simulink model "Servosistema_integrador_realimentacao"  (R2023b)
settings: Solver=FixedStepAuto  StartTime=0.0  StopTime=5  FixedStep=T  RelTol=1e-3
model workspace (MAT data in the model file):
  B = 0.0928995746863
  J = 0.56
  K = [0.48 -97.1871]
  Kf = 1.9158692362
  Ki = -97.6271
  Ko = [133.0634; 1.89971]
  L = 0.0014
  R = 0.08
  T = 0.00175
  Te = 0.0175
  Tm = 6.02801468027
  Vn = 400
  m_A = [0.9  -2.39483654525; 0.00598709136312  0.999709688829]
  m_B = [0; -0.003125]
  m_C = [0 1]
settings Model: Creator=USER  LastModifiedBy=lpds

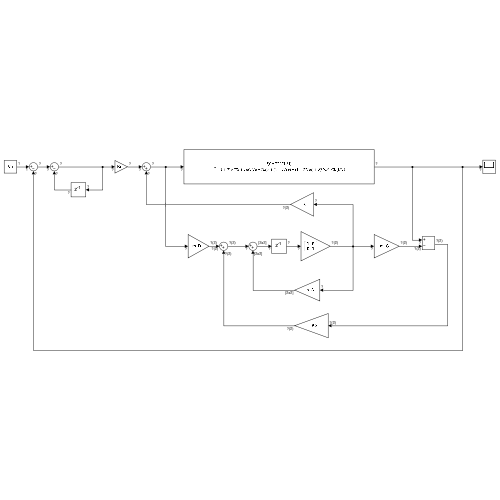
[thumbnail: Simulink's stored preview of the top-level diagram]
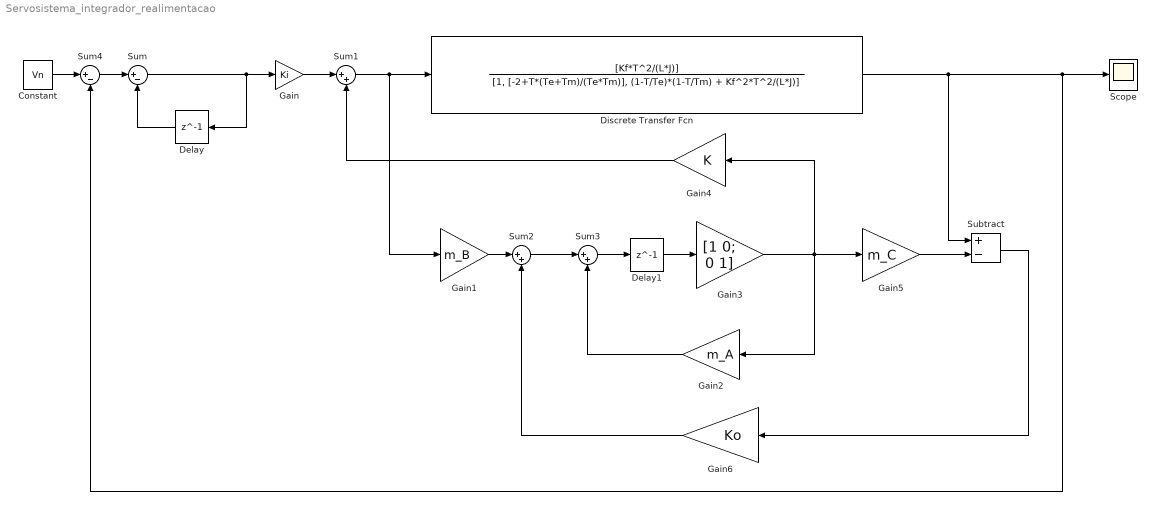
== system Servosistema_integrador_realimentacao ==
  Constant : Constant  Value=Vn
  Delay : Delay  DelayLength=1
  Delay1 : Delay  DelayLength=1  InitialCondition=0
  Discrete Transfer Fcn : DiscreteTransferFcn  Numerator=[Kf*T^2/(L*J)]  Denominator=[1, [-2+T*(Te+Tm)/(Te*Tm)], (1-T/Te)*(1-T/Tm) + Kf^2*T^2/(L*J)]
  Gain : Gain  Gain=Ki
  Gain1 : Gain  Gain=m_B
  Gain2 : Gain  Gain=m_A
  Gain3 : Gain  Gain=[1 0; 0 1]
  Gain4 : Gain  Gain=K
  Gain5 : Gain  Gain=m_C
  Gain6 : Gain  Gain=Ko
  Scope : Scope
  Subtract : Sum  Inputs=+-
  Sum : Sum  Inputs=|+-
  Sum1 : Sum  Inputs=|++
  Sum2 : Sum  Inputs=|++
  Sum3 : Sum  Inputs=|++
  Sum4 : Sum  Inputs=|+-
  wires:
  Sum/1 -> Delay/1, Gain/1
  Delay/1 -> Sum/2
  Gain/1 -> Sum1/1
  Sum1/1 -> Gain1/1, Discrete Transfer Fcn/1
  Discrete Transfer Fcn/1 -> Scope/1, Sum4/2, Subtract/1
  Gain1/1 -> Sum2/1
  Sum2/1 -> Sum3/1
  Gain2/1 -> Sum3/2
  Gain3/1 -> Gain4/1, Gain5/1, Gain2/1
  Gain4/1 -> Sum1/2
  Gain5/1 -> Subtract/2
  Subtract/1 -> Gain6/1
  Gain6/1 -> Sum2/2
  Constant/1 -> Sum4/1
  Sum4/1 -> Sum/1
  Sum3/1 -> Delay1/1
  Delay1/1 -> Gain3/1
